simulink model "Subsystem"  (R2020b)
settings: Solver=VariableStepAuto  StartTime=0.0  StopTime=10.0  RelTol=1e-3
settings Model: Creator=Shantam Garg  LastModifiedBy=Shantam Garg
settings DataIOCC: SaveOutput=off  SaveTime=off

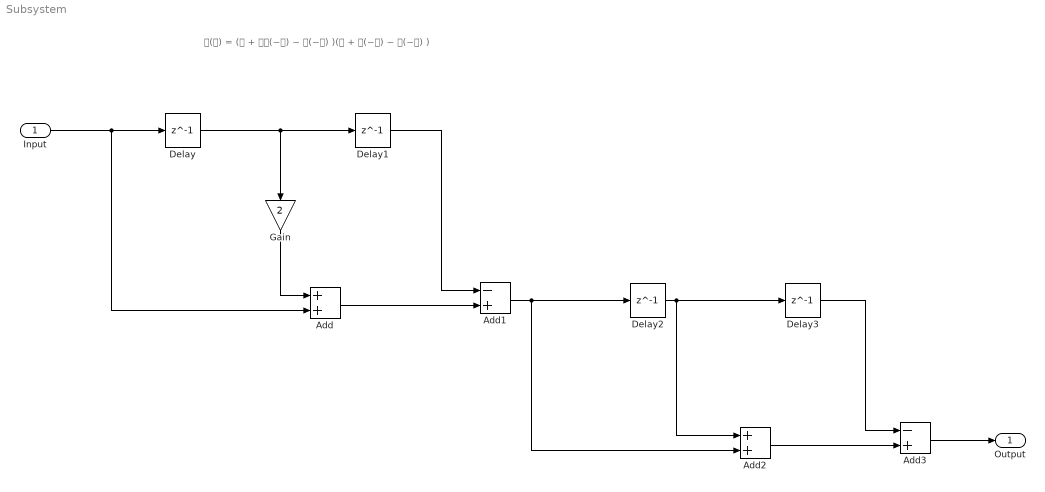
== system Subsystem ==
  note: 𝐇(𝐳) = (𝟏 + 𝟐𝐳(−𝟏) − 𝐳(−𝟐) )(𝟏 + 𝐳(−𝟏) − 𝐳(−𝟐) )
  "Input  " : Inport  OutDataTypeStr=double  PortDimensions=1  SampleTime=[0,1]
  Add : Sum
  Add1 : Sum  Inputs=-+
  Add2 : Sum
  Add3 : Sum  Inputs=-+
  Delay{,1..3} (4 alike) : Delay  DelayLength=1
  Gain : Gain  Gain=2
  Output : Outport  OutDataTypeStr=double  PortDimensions=1  SampleTime=[0,1]
  wires:
  Add2/1 -> Add3/2
  Delay1/1 -> Add1/1
  Delay2/1 -> Delay3/1, Add2/1
  "Input  "/1 -> Delay/1, Add/2
  Gain/1 -> Add/1
  Add1/1 -> Delay2/1, Add2/2
  Delay/1 -> Gain/1, Delay1/1
  Delay3/1 -> Add3/1
  Add/1 -> Add1/2
  Add3/1 -> Output/1
